simulink model "stabilitate3"  (R2024a)
settings: Solver=VariableStepAuto  StartTime=0.0  StopTime=1000  RelTol=1e-3
values from neighbouring files (symbols this model uses):
  ki = 3    [parametrii.m]
  kp = 4    [parametrii.m]
settings Model: Creator=paulhondola  LastModifiedBy=paulhondola

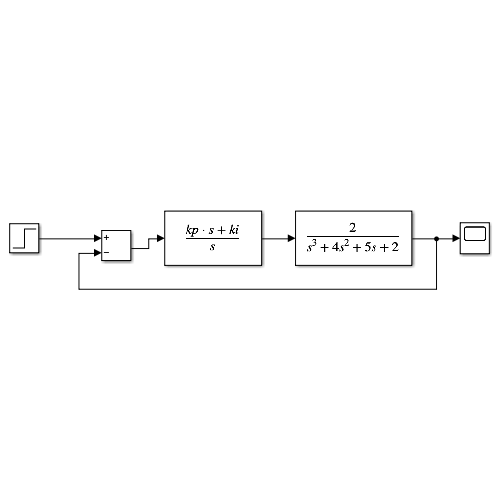
[thumbnail: Simulink's stored preview of the top-level diagram]
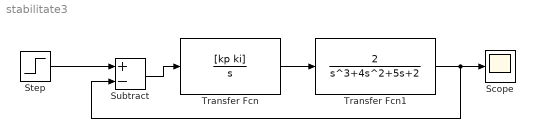
== system stabilitate3 ==
  Scope : Scope
  Step : Step  After=5  SampleTime=0
  Subtract : Sum  Inputs=+-
  Transfer Fcn : TransferFcn  Numerator=[kp ki]  Denominator=[1 0]
  Transfer Fcn1 : TransferFcn  Numerator=[2]  Denominator=[1 4 5 2]
  wires:
  Transfer Fcn/1 -> Transfer Fcn1/1
  Transfer Fcn1/1 -> Subtract/2, Scope/1
  Subtract/1 -> Transfer Fcn/1
  Step/1 -> Subtract/1
